simulink model "Auxilliary_Data_Filtering"  (R2022a)
settings: Solver=FixedStepDiscrete  StartTime=0.0  StopTime=10.0  FixedStep=0.01  RelTol=1e-3
settings Model: DataDictionary=VSM_Data_Dictionary.sldd  EnableAccessToBaseWorkspace=off  DVExtractedSubsystem=Auxilliary_Data_Filtering  Creator=jamesbond  LastModifiedBy=jamesbond
settings OptimizationCC: DefaultParameterBehavior=Inlined  EnhancedBackFolding=on  PassReuseOutputArgsAs=Individual arguments  ZeroExternalMemoryAtStartup=off  ZeroInternalMemoryAtStartup=off  OptimizeBlockOrder=speed  DifferentSizesBufferReuse=on  OptimizationCustomize=off  EfficientTunableParamExpr=on
settings DebuggingCC: SignalInfNanChecking=error  SignalRangeChecking=warning  CheckMatrixSingularityMsg=error  IntegerOverflowMsg=none  ParameterOverflowMsg=none  ParameterTunabilityLossMsg=error  FrameProcessingCompatibilityMsg=none  BusObjectLabelMismatch=error  ModelReferenceVersionMismatchMessage=warning  ModelReferenceIOMismatchMessage=warning  IntegerSaturationMsg=none
settings SFSimCC: MATLABDynamicMemAlloc=off
settings RTWCC: SystemTargetFile=ert.tlc  TemplateMakefile=ert_default_tmf  GenerateReport=on
settings CodeAppCC: ForceParamTrailComments=on  IgnoreCustomStorageClasses=off  OperatorAnnotations=on  SimulinkDataObjDesc=on  SFDataObjDesc=on  InsertBlockDesc=on
settings ERTTargetCC: TargetLangStandard=C99 (ISO)  GenerateSampleERTMain=on  InlinedParameterPlacement=NonHierarchical  ERTCustomFileTemplate=example_file_process.tlc
settings ConfigComp: DVModelCoverageObjectives=MCDC  DVTestSuiteOptimization=Auto  DVDetectDeadLogic=on  DVDetectOutOfBounds=on  DVModelReferenceHarness=on  DVHarnessSource=Signal Editor

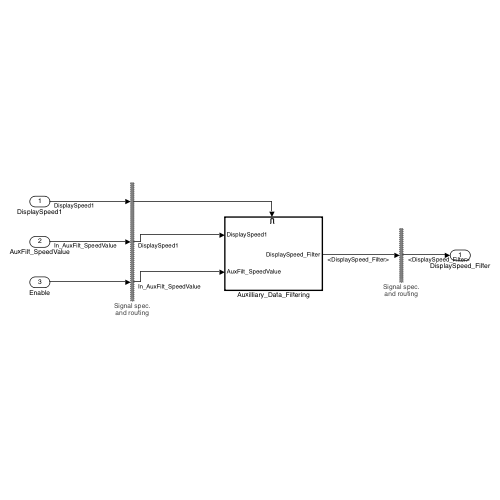
[thumbnail: Simulink's stored preview of the top-level diagram]
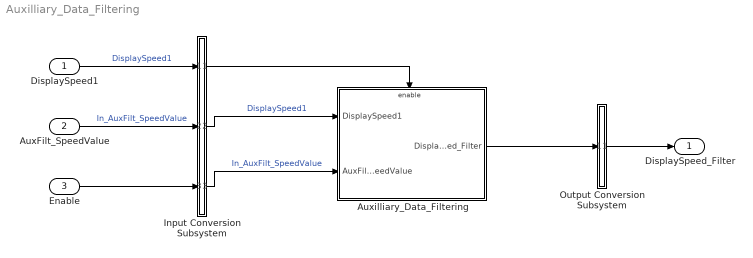
== system Auxilliary_Data_Filtering ==
  DisplaySpeed1 : Inport  OutDataTypeStr=fixdt('ufix16_Sp01')  PortDimensions=[1]  SampleTime=0.01  Interpolate=off
  AuxFilt_SpeedValue : Inport  Port=2  OutMin=1  OutMax=3  OutDataTypeStr=uint8  PortDimensions=[1]  SampleTime=0.01  Interpolate=off
  Enable : Inport  Port=3  OutDataTypeStr=boolean  PortDimensions=[1]  SampleTime=0.01  Interpolate=off
  Auxilliary_Data_Filtering : Subsystem  TreatAsAtomicUnit=on
  Input Conversion Subsystem : Subsystem  Tag=__SLT_ICS__  Description=|
      | Signal spec.
      | and routing
      settings: AttributesFormatString=%<Description>
  Output Conversion Subsystem : Subsystem  Tag=__SLT_OCS__  Description=|
      | Signal spec.
      | and routing
      settings: AttributesFormatString=%<Description>
  DisplaySpeed_Filter : Outport
  wires:
  DisplaySpeed1/1 -> Input Conversion Subsystem/1(Inport_1)  "DisplaySpeed1"
  AuxFilt_SpeedValue/1 -> Input Conversion Subsystem/2(Inport_2)  "In_AuxFilt_SpeedValue"
  Enable/1 -> Input Conversion Subsystem/3(Inport_3)
  Output Conversion Subsystem/1(Outport_1) -> DisplaySpeed_Filter/1
  Input Conversion Subsystem/1(Outport_3) -> Auxilliary_Data_Filtering/Enable
  Input Conversion Subsystem/2(Outport_1) -> Auxilliary_Data_Filtering/1(DisplaySpeed1)  "DisplaySpeed1"
  Input Conversion Subsystem/3(Outport_2) -> Auxilliary_Data_Filtering/2(AuxFilt_SpeedValue)  "In_AuxFilt_SpeedValue"
  Auxilliary_Data_Filtering/1(DisplaySpeed_Filter) -> Output Conversion Subsystem/1(Inport_1)

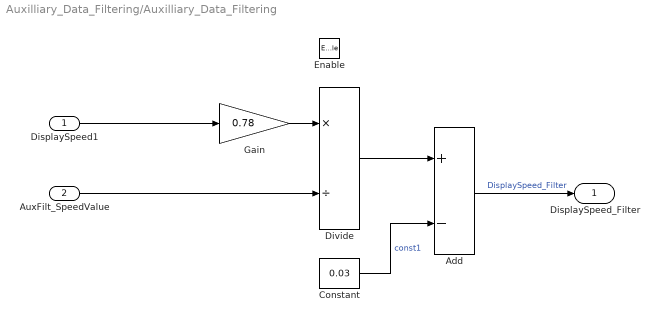
== system Auxilliary_Data_Filtering/Auxilliary_Data_Filtering ==
  DisplaySpeed1 : Inport  OutDataTypeStr=fixdt(0,16,0.01,0)  PortDimensions=1  SampleTime=0.01
  AuxFilt_SpeedValue : Inport  Port=2
  Enable : EnablePort
  Add : Sum  Inputs=+-  AccumDataTypeStr=fixdt(0,16,0.01,0)  OutDataTypeStr=fixdt(0,16,0.01,0)
  Constant : Constant  Value=0.03  OutMin=0.03  OutMax=0.03  OutDataTypeStr=fixdt(0,16,0.01,0)
  Divide : Product  Inputs=*/  OutDataTypeStr=fixdt(0,16,0.01,0)
  Gain : Gain  Gain=0.78  ParamMin=0.78  ParamMax=0.78  ParamDataTypeStr=fixdt(0,16,0.01,0)  OutDataTypeStr=fixdt(0,16,0.01,0)
  DisplaySpeed_Filter : Outport  OutDataTypeStr=fixdt(0,16,0.01,0)  PortDimensions=1  SampleTime=0.01
  wires:
  Divide/1 -> Add/1
  AuxFilt_SpeedValue/1 -> Divide/2
  DisplaySpeed1/1 -> Gain/1
  Constant/1 -> Add/2  "const1"
  Add/1 -> DisplaySpeed_Filter/1  "DisplaySpeed_Filter"
  Gain/1 -> Divide/1

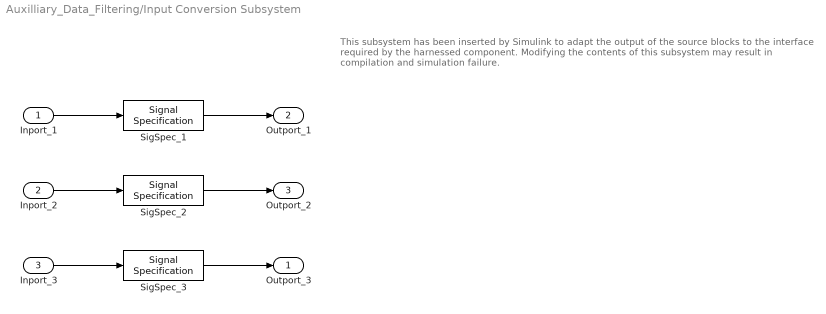
== system Auxilliary_Data_Filtering/Input Conversion Subsystem ==
  note: This subsystem has been inserted by Simulink to adapt the output of the source blocks to the interface required by the harnessed component.
      |  Modifying the contents of this subsystem may result in compilation and simulation failure.
  Inport_1 : Inport
  Inport_2 : Inport  Port=2
  Inport_3 : Inport  Port=3
  SigSpec_1 : SignalSpecification  OutDataTypeStr=fixdt('ufix16_Sp01')  Dimensions=[1]  SampleTime=0.01
  SigSpec_2 : SignalSpecification  OutDataTypeStr=uint8  Dimensions=[1]  SampleTime=0.01
  SigSpec_3 : SignalSpecification  OutDataTypeStr=boolean  Dimensions=[1]  SampleTime=0.01
  Outport_3 : Outport
  Outport_1 : Outport  Port=2
  Outport_2 : Outport  Port=3
  wires:
  SigSpec_1/1 -> Outport_1/1
  Inport_1/1 -> SigSpec_1/1
  SigSpec_2/1 -> Outport_2/1
  Inport_2/1 -> SigSpec_2/1
  SigSpec_3/1 -> Outport_3/1
  Inport_3/1 -> SigSpec_3/1

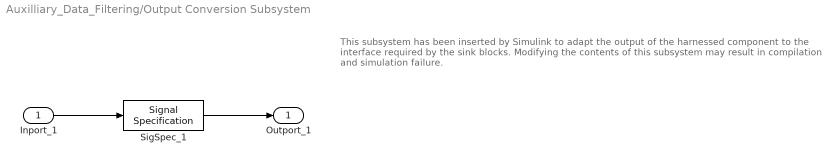
== system Auxilliary_Data_Filtering/Output Conversion Subsystem ==
  note: This subsystem has been inserted by Simulink to adapt the output of the harnessed component to the interface required by the sink blocks.
      |  Modifying the contents of this subsystem may result in compilation and simulation failure.
  Inport_1 : Inport
  SigSpec_1 : SignalSpecification  OutDataTypeStr=fixdt('ufix16_Sp01')  Dimensions=[1]  SampleTime=0.01
  Outport_1 : Outport
  wires:
  Inport_1/1 -> SigSpec_1/1
  SigSpec_1/1 -> Outport_1/1
